simulink model "ClosedLoopStimXpcTarget_1NSP"  (R2016b)
settings: Solver=FixedStepDiscrete  StartTime=0.0  StopTime=inf  FixedStep=sCoreParams.core.stepPeriod  RelTol=1e-3  EnableMultiTasking=on
values from neighbouring files (symbols this model uses):
  sCoreParams = InitCoreParams_Dependent(sCoreParams)    [initializationScript.m]
libraries: dspswit3 x7, slrtlib x5
settings Model: DataTypeOverride=Double  MinMaxOverflowLogging=ForceOff  Creator=rzelmann  LastModifiedBy=rzelmann
settings SolverCC: EnableConcurrentExecution=on  ConcurrentTasks=on
settings DataIOCC: SaveFormat=StructureWithTime
settings OptimizationCC: DefaultParameterBehavior=Inlined  EfficientFloat2IntCast=on  LifeSpan=inf
settings DebuggingCC: UniqueDataStoreMsg=error  StrictBusMsg=ErrorOnBusTreatedAsVector  SFUnexpectedBacktrackingDiag=warning  SFNoUnconditionalDefaultTransitionDiag=warning  SFExecutionAtInitializationDiag=none
settings HardwareCC: ProdBitPerPointer=32  ProdBitPerSizeT=32  ProdBitPerPtrDiffT=32  ProdLargestAtomicFloat=None  ProdWordSize=32  ProdLongLongMode=on  ProdHWDeviceType=Generic->32-bit x86 compatible
settings ModelReferenceCC: ModelReferenceNumInstancesAllowed=Single
settings RTWCC: SystemTargetFile=slrt.tlc  TLCOptions="-axPCMaxOverloads=30            -axPCOverLoadLen=2 -axPCStartupFlag=5"  TemplateMakefile=slrt_default_tmf  Description=Simulink Real-Time  RTWCompilerOptimization=on
settings CodeAppCC: MaxIdLength=63
settings TargetCC: CodeReplacementLibrary=XPC_BLAS  ParMdlRefBuildCompliant=on  ConcurrentExecutionCompliant=on  GeneratePreprocessorConditionals=Use local settings  MatFileLogging=on  MATLABClassNameForMDSCustomization=xpcAperiodicCustomization
settings ConfigComp: CovMetricSettings=dw  CovHtmlReporting=on  CovSaveCumulativeToWorkspaceVar=on  CovSaveSingleToWorkspaceVar=on  CovExternalEMLEnable=off

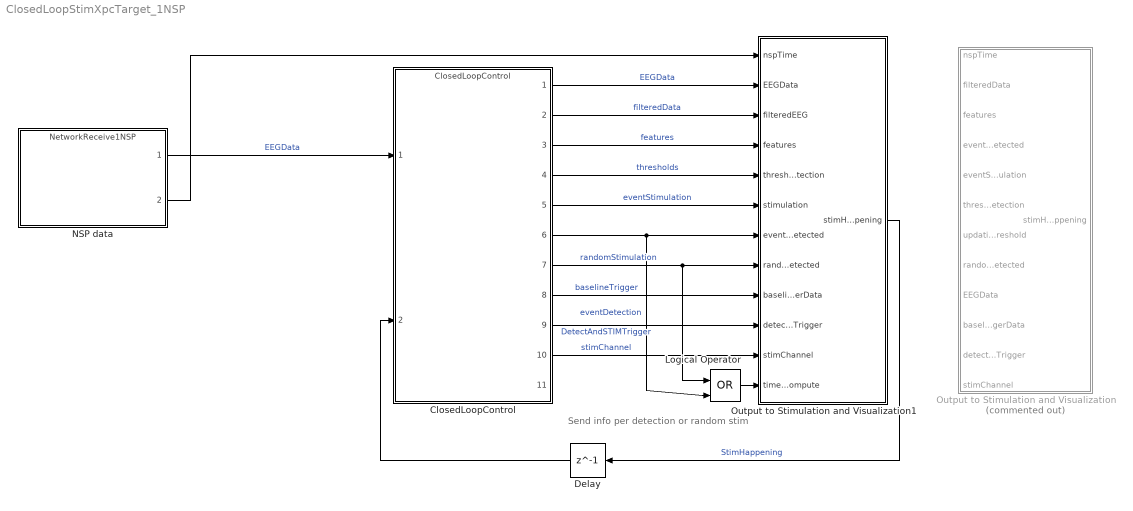
== system ClosedLoopStimXpcTarget_1NSP ==
  note: Send info per detection or random stim
  ClosedLoopControl : ModelReference  ModelNameDialog=ClosedLoopControl  SimulationMode=Normal  ModelReferenceVersion=1.712
  Delay : Delay  DelayLength=1  InitialCondition=0  InputProcessing=Columns as channels (frame based)  SampleTime=sCoreParams.core.stepPeriod
  Logical Operator : Logic  Operator=OR  IconShape=distinctive  AllPortsSameDT=off  OutDataTypeStr=boolean
  NSP data : ModelReference  ModelNameDialog=NetworkReceive1NSP.slx  SimulationMode=Normal  ModelReferenceVersion=1.191
  Output to Stimulation and Visualization : Subsystem  Commented=on
  Output to Stimulation and Visualization1 : Subsystem
  wires:
  Output to Stimulation and Visualization1/1(stimHappening) -> Delay/1  "StimHappening"
  NSP data/1 -> ClosedLoopControl/1  "EEGData"
  ClosedLoopControl/1 -> Output to Stimulation and Visualization1/2(EEGData)  "EEGData"
  NSP data/2 -> Output to Stimulation and Visualization1/1(nspTime)
  ClosedLoopControl/4 -> Output to Stimulation and Visualization1/5(thresholdUsedInDetection)  "thresholds"
  ClosedLoopControl/6 -> Logical Operator/2, Output to Stimulation and Visualization1/7(eventDetected)  "eventDetection"
  ClosedLoopControl/8 -> Output to Stimulation and Visualization1/9(baselineTriggerData)  "baselineTrigger"
  ClosedLoopControl/9 -> Output to Stimulation and Visualization1/10(detectStimTrigger)  "DetectAndSTIMTrigger"
  ClosedLoopControl/10 -> Output to Stimulation and Visualization1/11(stimChannel)  "stimChannel"
  Delay/1 -> ClosedLoopControl/2
  ClosedLoopControl/7 -> Logical Operator/1, Output to Stimulation and Visualization1/8(randomDetected)  "randomStimulation"
  ClosedLoopControl/5 -> Output to Stimulation and Visualization1/6(stimulation)  "eventStimulation"
  ClosedLoopControl/3 -> Output to Stimulation and Visualization1/4(features)  "features"
  ClosedLoopControl/2 -> Output to Stimulation and Visualization1/3(filteredEEG)  "filteredData"
  Logical Operator/1 -> Output to Stimulation and Visualization1/12(timeToCompute)

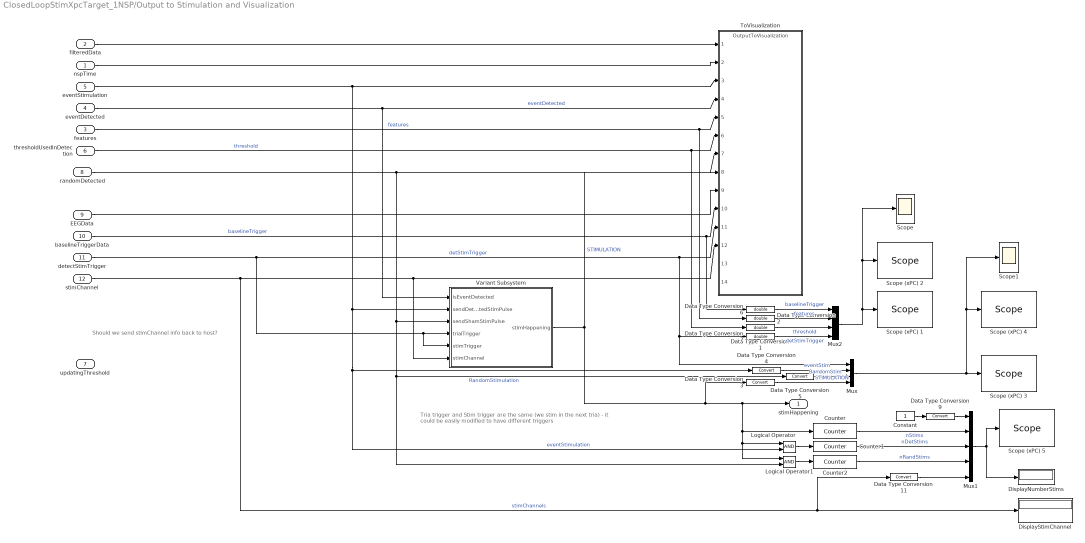
== system ClosedLoopStimXpcTarget_1NSP/Output to Stimulation and Visualization ==
  note: Should we send stimChannel info back to host?
  note: Tria trigger and Stim trigger are the same (we stim in the next tria)
      | - it could be easily modified to have different triggers
  nspTime : Inport
  filteredData : Inport  Port=2
  features : Inport  Port=3
  eventDetected : Inport  Port=4
  eventStimulation : Inport  Port=5
  thresholdUsedInDetection : Inport  Port=6
  updatingThreshold : Inport  Port=7
  randomDetected : Inport  Port=8
  EEGData : Inport  Port=9
  baselineTriggerData : Inport  Port=10  OutDataTypeStr=int32
  detectStimTrigger : Inport  Port=11  OutDataTypeStr=int32
  stimChannel : Inport  Port=12
  Constant : Constant  OutDataTypeStr=int32
  Counter : dspswit3/Counter  Direction=Up  CountEvent=Rising edge  CounterSize=User defined  MaxCount=1024  InitialCount=0  Output=Count  HitValue=32  ResetInput=off  SamplesPerFrame=1  Ts=1  CntDtype=int32  HitDtype=Logical
  Counter1 : dspswit3/Counter  Direction=Up  CountEvent=Rising edge  CounterSize=User defined  MaxCount=1024  InitialCount=0  Output=Count  HitValue=32  ResetInput=off  SamplesPerFrame=1  Ts=1  CntDtype=int32  HitDtype=Logical
  Counter2 : dspswit3/Counter  Direction=Up  CountEvent=Rising edge  CounterSize=User defined  MaxCount=1024  InitialCount=0  Output=Count  HitValue=32  ResetInput=off  SamplesPerFrame=1  Ts=1  CntDtype=int32  HitDtype=Logical
  Data Type Conversion{1..2,6..7} (4 alike) : DataTypeConversion  OutDataTypeStr=double
  Data Type Conversion{3..5,9,11} (5 alike) : DataTypeConversion
  DisplayNumberStims : Display
      settings: Format=decimal (Stored Integer)
  DisplayStimChannel : Display
  Logical Operator : Logic  IconShape=distinctive  AllPortsSameDT=off  OutDataTypeStr=boolean
  Logical Operator1 : Logic  IconShape=distinctive  AllPortsSameDT=off  OutDataTypeStr=boolean
  Mux : Mux
  Mux1 : Mux  Inputs=5
  Mux2 : Mux
  Scope : Scope
  Scope (xPC) 1 : slrtlib/Displays and Logging/Scope   scopeno=3  scopetype=Target  autostart=on  viewmode=Graphical sliding  formatstr='%15.6f'  grid=on  ylimits=[0,0]  nosamples=1000  noprepostsamples=0  interleave=1  triggermode=FreeRun  triggersignal=1  trigsignalfromport=on  triggerlevel=0.0  triggerslope=Rising  triggerscope=1  triggersample=0  filename=data.dat  mode=Lazy  writesize=512  autorestart=off  dynamicfilemode=off  maxwritefilesize=512*1024^2
  Scope (xPC) 2 : slrtlib/Displays and Logging/Scope   scopeno=2  scopetype=File  autostart=on  viewmode=Graphical redraw  formatstr='%15.6f'  grid=on  ylimits=[0,0]  nosamples=1000  noprepostsamples=-10  interleave=1  triggermode=FreeRun  triggersignal=1  trigsignalfromport=on  triggerlevel=0.0  triggerslope=Rising  triggerscope=1  triggersample=0  filename=featTh.dat  mode=Lazy  writesize=512  autorestart=off  dynamicfilemode=off  maxwritefilesize=512*1024^2
  Scope (xPC) 3 : slrtlib/Displays and Logging/Scope   scopeno=5  scopetype=Target  autostart=on  viewmode=Graphical sliding  formatstr='%15.6f'  grid=on  ylimits=[0,0]  nosamples=1000  noprepostsamples=0  interleave=1  triggermode=FreeRun  triggersignal=1  trigsignalfromport=on  triggerlevel=0.0  triggerslope=Rising  triggerscope=1  triggersample=0  filename=data.dat  mode=Lazy  writesize=512  autorestart=off  dynamicfilemode=off  maxwritefilesize=512*1024^2
  Scope (xPC) 4 : slrtlib/Displays and Logging/Scope   scopeno=4  scopetype=File  autostart=on  viewmode=Graphical redraw  formatstr='%15.6f'  grid=on  ylimits=[0,0]  nosamples=1000  noprepostsamples=-10  interleave=1  triggermode=FreeRun  triggersignal=1  trigsignalfromport=on  triggerlevel=0.0  triggerslope=Rising  triggerscope=1  triggersample=0  filename=detStim.dat  mode=Lazy  writesize=512  autorestart=off  dynamicfilemode=off  maxwritefilesize=512*1024^2
  Scope (xPC) 5 : slrtlib/Displays and Logging/Scope   scopeno=7  scopetype=Target  autostart=on  viewmode=Numerical  formatstr='%d'  grid=on  ylimits=[0,0]  nosamples=1000  noprepostsamples=0  interleave=1  triggermode=FreeRun  triggersignal=1  trigsignalfromport=on  triggerlevel=0.0  triggerslope=Rising  triggerscope=1  triggersample=0  filename=data.dat  mode=Lazy  writesize=512  autorestart=off  dynamicfilemode=off  maxwritefilesize=512*1024^2
  Scope1 : Scope
  ToVisualization : ModelReference  ModelNameDialog=OutputToVisualization  SimulationMode=Normal  ModelReferenceVersion=1.265
  Variant Subsystem : Subsystem  Variant=on
  stimHappening : Outport  OutDataTypeStr=boolean  SampleTime=sCoreParams.core.stepPeriod
  wires:
  eventDetected/1 -> Variant Subsystem/1(isEventDetected), ToVisualization/4  "eventDetected"
  nspTime/1 -> ToVisualization/2
  randomDetected/1 -> Logical Operator1/2, Data Type Conversion5/1, Variant Subsystem/3(sendShamStimPulse), ToVisualization/7  "RandomStimulation"
  Variant Subsystem/1(stimHappening) -> ToVisualization/8, Data Type Conversion3/1, Logical Operator1/1, Logical Operator/1, Counter/1, stimHappening/1  "STIMULATION"
  eventStimulation/1 -> ToVisualization/3, Variant Subsystem/2(sendDetectedStimPulse), Logical Operator/2, Data Type Conversion4/1  "eventStimulation"
  filteredData/1 -> ToVisualization/1
  EEGData/1 -> ToVisualization/9
  features/1 -> Data Type Conversion2/1, ToVisualization/5  "features"
  thresholdUsedInDetection/1 -> Data Type Conversion1/1, ToVisualization/6  "threshold"
  Data Type Conversion3/1 -> Mux/4  "STIMULATION"
  Data Type Conversion4/1 -> Mux/2  "eventStim"
  Mux2/1 -> Scope/1, Scope (xPC) 2/1, Scope (xPC) 1/1
  Mux/1 -> Scope1/1, Scope (xPC) 4/1, Scope (xPC) 3/1
  Data Type Conversion5/1 -> Mux/3  "RandomStim"
  baselineTriggerData/1 -> Data Type Conversion6/1, ToVisualization/10  "baselineTrigger"
  Data Type Conversion1/1 -> Mux2/3  "threshold"
  Data Type Conversion2/1 -> Mux2/2  "features"
  Data Type Conversion6/1 -> Mux2/1  "baselineTrigger"
  detectStimTrigger/1 -> Variant Subsystem/5(stimTrigger), Variant Subsystem/4(trialTrigger), Mux/1, Data Type Conversion7/1, ToVisualization/11  "detStimTrigger"
  Data Type Conversion7/1 -> Mux2/4  "detStimTrigger"
  stimChannel/1 -> Variant Subsystem/6(stimChannel), ToVisualization/12, DisplayStimChannel/1, Data Type Conversion11/1  "stimChannels"
  Mux1/1 -> DisplayNumberStims/1, Scope (xPC) 5/1
  Counter1/1 -> Mux1/3  "nDetStims"
  Counter2/1 -> Mux1/4  "nRandStims"
  Data Type Conversion11/1 -> Mux1/5
  Counter/1 -> Mux1/2  "nStims"
  Constant/1 -> Data Type Conversion9/1
  Data Type Conversion9/1 -> Mux1/1
  Logical Operator/1 -> Counter1/1
  Logical Operator1/1 -> Counter2/1

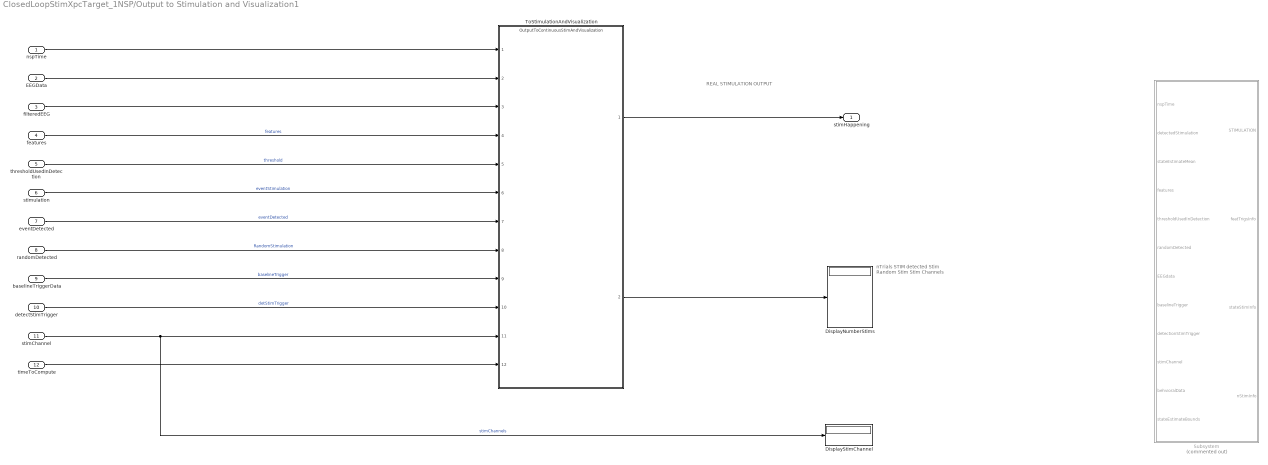
== system ClosedLoopStimXpcTarget_1NSP/Output to Stimulation and Visualization1 ==
  note: nTrials
      | STIM
      | detected Stim
      | Random Stim
      | Stim Channels
  note: REAL STIMULATION OUTPUT
  nspTime : Inport
  EEGData : Inport  Port=2
  filteredEEG : Inport  Port=3
  features : Inport  Port=4
  thresholdUsedInDetection : Inport  Port=5
  stimulation : Inport  Port=6
  eventDetected : Inport  Port=7
  randomDetected : Inport  Port=8
  baselineTriggerData : Inport  Port=9  OutDataTypeStr=int32
  detectStimTrigger : Inport  Port=10  OutDataTypeStr=int32
  stimChannel : Inport  Port=11
  timeToCompute : Inport  Port=12  OutDataTypeStr=boolean
  DisplayNumberStims : Display
      settings: Format=decimal (Stored Integer)
  DisplayStimChannel : Display
  Subsystem : Subsystem  Commented=on
  ToStimulationAndVisualization : ModelReference  ModelNameDialog=OutputToContinuousStimAndVisualization.slx  SimulationMode=Normal  ModelReferenceVersion=1.305
  stimHappening : Outport  OutDataTypeStr=boolean  SampleTime=sCoreParams.core.stepPeriod
  wires:
  stimChannel/1 -> ToStimulationAndVisualization/11, DisplayStimChannel/1  "stimChannels"
  ToStimulationAndVisualization/2 -> DisplayNumberStims/1
  ToStimulationAndVisualization/1 -> stimHappening/1
  nspTime/1 -> ToStimulationAndVisualization/1
  EEGData/1 -> ToStimulationAndVisualization/2
  filteredEEG/1 -> ToStimulationAndVisualization/3
  features/1 -> ToStimulationAndVisualization/4  "features"
  thresholdUsedInDetection/1 -> ToStimulationAndVisualization/5  "threshold"
  stimulation/1 -> ToStimulationAndVisualization/6  "eventStimulation"
  detectStimTrigger/1 -> ToStimulationAndVisualization/10  "detStimTrigger"
  baselineTriggerData/1 -> ToStimulationAndVisualization/9  "baselineTrigger"
  timeToCompute/1 -> ToStimulationAndVisualization/12
  eventDetected/1 -> ToStimulationAndVisualization/7  "eventDetected"
  randomDetected/1 -> ToStimulationAndVisualization/8  "RandomStimulation"

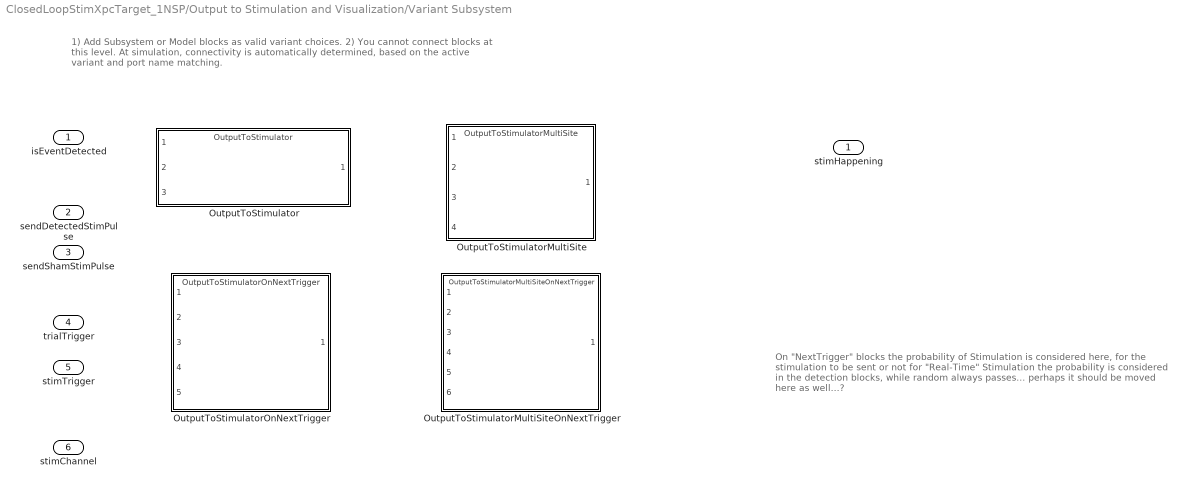
== system ClosedLoopStimXpcTarget_1NSP/Output to Stimulation and Visualization/Variant Subsystem ==
  note: On "NextTrigger" blocks the probability of Stimulation is considered here,
      | for the stimulation to be sent or not
      | for "Real-Time" Stimulation the probability is considered in the detection blocks,
      | while random always passes... perhaps it should be moved here as well...?
  note: 1) Add Subsystem or Model blocks as valid variant choices.
      | 2) You cannot connect blocks at this level. At simulation, connectivity is automatically
      | determined, based on the active variant and port name matching.
  isEventDetected : Inport
  sendDetectedStimPulse : Inport  Port=2
  sendShamStimPulse : Inport  Port=3
  trialTrigger : Inport  Port=4
  stimTrigger : Inport  Port=5
  stimChannel : Inport  Port=6  OutDataTypeStr=int32
  OutputToStimulator : ModelReference  ModelNameDialog=OutputToStimulator  SimulationMode=Normal  VariantControl=variantParams_STIMULATION_REALTIME  ModelReferenceVersion=1.34
  OutputToStimulatorMultiSite : ModelReference  ModelNameDialog=OutputToStimulatorMultiSite.slx  SimulationMode=Normal  VariantControl=variantParams_STIMULATION_MULTISITE_REALTIME  ModelReferenceVersion=1.46
  OutputToStimulatorMultiSiteOnNextTrigger : ModelReference  ModelNameDialog=OutputToStimulatorMultiSiteOnNextTrigger.slx  SimulationMode=Normal  VariantControl=variantParams_STIMULATION_MULTISITE_NEXTTRIGGER  ModelReferenceVersion=1.77
  OutputToStimulatorOnNextTrigger : ModelReference  ModelNameDialog=OutputToStimulatorOnNextTrigger  SimulationMode=Normal  VariantControl=variantParams_STIMULATION_ONNEXTTRIGGER  ModelReferenceVersion=1.85
  stimHappening : Outport

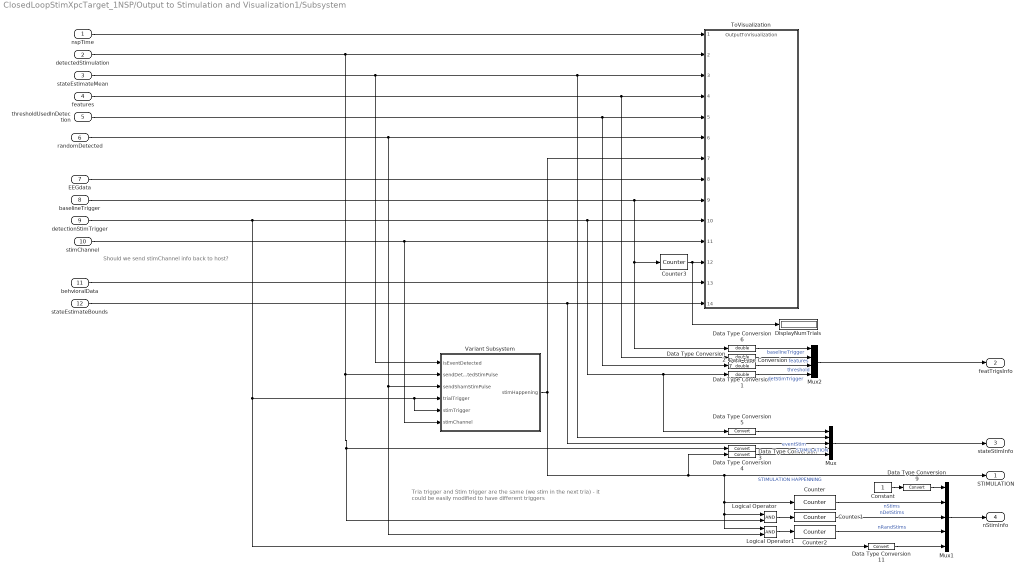
== system ClosedLoopStimXpcTarget_1NSP/Output to Stimulation and Visualization1/Subsystem ==
  note: Should we send stimChannel info back to host?
  note: Tria trigger and Stim trigger are the same (we stim in the next tria)
      | - it could be easily modified to have different triggers
  nspTime : Inport
  detectedStimulation : Inport  Port=2
  stateEstimateMean : Inport  Port=3
  features : Inport  Port=4
  thresholdUsedInDetection : Inport  Port=5
  randomDetected : Inport  Port=6
  EEGdata : Inport  Port=7
  baselineTrigger : Inport  Port=8
  detectionStimTrigger : Inport  Port=9
  stimChannel : Inport  Port=10
  behvioralData : Inport  Port=11
  stateEstimateBounds : Inport  Port=12
  Constant : Constant  OutDataTypeStr=int32
  Counter : dspswit3/Counter  Direction=Up  CountEvent=Rising edge  CounterSize=User defined  MaxCount=1024  InitialCount=0  Output=Count  HitValue=32  ResetInput=off  SamplesPerFrame=1  Ts=1  CntDtype=int32  HitDtype=Logical
  Counter1 : dspswit3/Counter  Direction=Up  CountEvent=Rising edge  CounterSize=User defined  MaxCount=1024  InitialCount=0  Output=Count  HitValue=32  ResetInput=off  SamplesPerFrame=1  Ts=1  CntDtype=int32  HitDtype=Logical
  Counter2 : dspswit3/Counter  Direction=Up  CountEvent=Rising edge  CounterSize=User defined  MaxCount=1024  InitialCount=0  Output=Count  HitValue=32  ResetInput=off  SamplesPerFrame=1  Ts=1  CntDtype=int32  HitDtype=Logical
  Counter3 : dspswit3/Counter  Direction=Up  CountEvent=Rising edge  CounterSize=User defined  MaxCount=1024  InitialCount=0  Output=Count  HitValue=32  ResetInput=off  SamplesPerFrame=1  Ts=1  CntDtype=double  HitDtype=Logical
  Data Type Conversion{1..2,6..7} (4 alike) : DataTypeConversion  OutDataTypeStr=double
  Data Type Conversion{3..5,9,11} (5 alike) : DataTypeConversion
  DisplayNumTrials : Display
  Logical Operator : Logic  IconShape=distinctive  AllPortsSameDT=off  OutDataTypeStr=boolean
  Logical Operator1 : Logic  IconShape=distinctive  AllPortsSameDT=off  OutDataTypeStr=boolean
  Mux : Mux  Inputs=5
  Mux1 : Mux  Inputs=5
  Mux2 : Mux
  ToVisualization : ModelReference  ModelNameDialog=OutputToVisualization  SimulationMode=Normal  ModelReferenceVersion=1.265
  Variant Subsystem : Subsystem  Variant=on
  STIMULATION : Outport
  featTrigsInfo : Outport  Port=2
  stateStimInfo : Outport  Port=3
  nStimInfo : Outport  Port=4
  wires:
  Counter1/1 -> Mux1/3  "nDetStims"
  nspTime/1 -> ToVisualization/1
  Data Type Conversion5/1 -> Mux/1
  behvioralData/1 -> ToVisualization/13
  Data Type Conversion11/1 -> Mux1/5
  detectedStimulation/1 -> Logical Operator/2, Data Type Conversion4/1, Variant Subsystem/2(sendDetectedStimPulse), ToVisualization/2
  Variant Subsystem/1(stimHappening) -> ToVisualization/7, Data Type Conversion3/1, STIMULATION/1, Logical Operator1/1, Logical Operator/1, Counter/1  "STIMULATION HAPPENNING"
  Logical Operator1/1 -> Counter2/1
  detectionStimTrigger/1 -> Data Type Conversion11/1, Variant Subsystem/5(stimTrigger), Variant Subsystem/4(trialTrigger), Data Type Conversion5/1, Data Type Conversion7/1, ToVisualization/10
  Counter3/1 -> DisplayNumTrials/1, ToVisualization/12
  Data Type Conversion6/1 -> Mux2/1  "baselineTrigger"
  Mux2/1 -> featTrigsInfo/1
  Data Type Conversion1/1 -> Mux2/3  "threshold"
  stimChannel/1 -> Variant Subsystem/6(stimChannel), ToVisualization/11
  baselineTrigger/1 -> Data Type Conversion6/1, Counter3/1, ToVisualization/9
  Logical Operator/1 -> Counter1/1
  Data Type Conversion9/1 -> Mux1/1
  stateEstimateMean/1 -> Variant Subsystem/1(isEventDetected), ToVisualization/3, Mux/2
  Counter/1 -> Mux1/2  "nStims"
  Data Type Conversion2/1 -> Mux2/2  "features"
  thresholdUsedInDetection/1 -> Data Type Conversion1/1, ToVisualization/5
  Data Type Conversion4/1 -> Mux/4  "eventStim"
  Mux1/1 -> nStimInfo/1
  Data Type Conversion7/1 -> Mux2/4  "detStimTrigger"
  Constant/1 -> Data Type Conversion9/1
  EEGdata/1 -> ToVisualization/8
  Counter2/1 -> Mux1/4  "nRandStims"
  Data Type Conversion3/1 -> Mux/5  "STIMULATION"
  features/1 -> Data Type Conversion2/1, ToVisualization/4
  Mux/1 -> stateStimInfo/1
  randomDetected/1 -> Logical Operator1/2, Variant Subsystem/3(sendShamStimPulse), ToVisualization/6
  stateEstimateBounds/1 -> Mux/3, ToVisualization/14

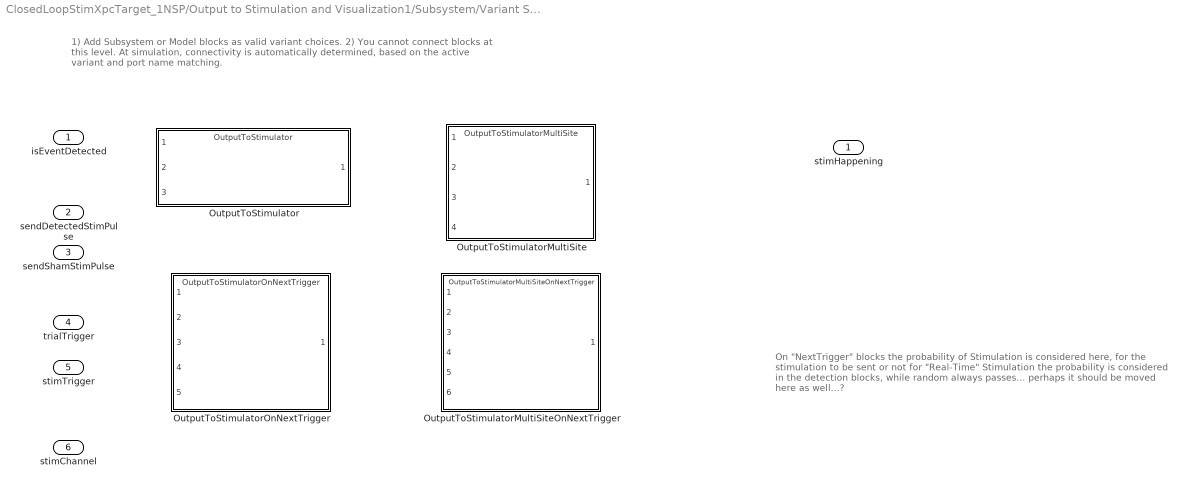
== system ClosedLoopStimXpcTarget_1NSP/Output to Stimulation and Visualization1/Subsystem/Variant Subsystem ==
  note: On "NextTrigger" blocks the probability of Stimulation is considered here,
      | for the stimulation to be sent or not
      | for "Real-Time" Stimulation the probability is considered in the detection blocks,
      | while random always passes... perhaps it should be moved here as well...?
  note: 1) Add Subsystem or Model blocks as valid variant choices.
      | 2) You cannot connect blocks at this level. At simulation, connectivity is automatically
      | determined, based on the active variant and port name matching.
  isEventDetected : Inport
  sendDetectedStimPulse : Inport  Port=2
  sendShamStimPulse : Inport  Port=3
  trialTrigger : Inport  Port=4
  stimTrigger : Inport  Port=5
  stimChannel : Inport  Port=6  OutDataTypeStr=int32
  OutputToStimulator : ModelReference  ModelNameDialog=OutputToStimulator  SimulationMode=Normal  VariantControl=variantParams_STIMULATION_REALTIME  ModelReferenceVersion=1.34
  OutputToStimulatorMultiSite : ModelReference  ModelNameDialog=OutputToStimulatorMultiSite.slx  SimulationMode=Normal  VariantControl=variantParams_STIMULATION_MULTISITE_REALTIME  ModelReferenceVersion=1.46
  OutputToStimulatorMultiSiteOnNextTrigger : ModelReference  ModelNameDialog=OutputToStimulatorMultiSiteOnNextTrigger.slx  SimulationMode=Normal  VariantControl=variantParams_STIMULATION_MULTISITE_NEXTTRIGGER  ModelReferenceVersion=1.77
  OutputToStimulatorOnNextTrigger : ModelReference  ModelNameDialog=OutputToStimulatorOnNextTrigger  SimulationMode=Normal  VariantControl=variantParams_STIMULATION_ONNEXTTRIGGER  ModelReferenceVersion=1.85
  stimHappening : Outport
